simulink model "Simulink"  (R2021a)
settings: Solver=FixedStepAuto  StartTime=0.0  StopTime=10.0  FixedStep=1e-3  RelTol=1e-3  EnableMultiTasking=on
undefined symbols (not defined in the file): D0, D1, D10, D11, D12, D13, D2, D3, D4, D5, D6, D7, D8, D9, PTA0, PTA1, PTA2, PTB23, PTB9, PTC16, PTC17, PTC2, PTC3, PTC4, PTD0, PTD1, PTD2, PTD3
libraries: frdmk64flib x19
settings Model: EnablePacing=on  PacingRate=0.250000  ExtModeTrigDuration=5  Creator=Arun Mistry  LastModifiedBy=Arun Mistry
settings OptimizationCC: EnhancedBackFolding=on  PassReuseOutputArgsAs=Individual arguments  ZeroExternalMemoryAtStartup=off  ZeroInternalMemoryAtStartup=off  MaxStackSize=64  OptimizeBlockOrder=speed  DifferentSizesBufferReuse=on  OptimizationCustomize=off  EfficientTunableParamExpr=on
settings DebuggingCC: ParameterTunabilityLossMsg=error
settings HardwareCC: ProdBitPerPointer=32  ProdBitPerSizeT=32  ProdBitPerPtrDiffT=32  ProdLargestAtomicInteger=Long  ProdLargestAtomicFloat=Double  ProdWordSize=32  ProdHWDeviceType=ARM Compatible->ARM Cortex
settings SFSimCC: MATLABDynamicMemAlloc=off
settings RTWCC: SystemTargetFile=ert.tlc  HardwareBoard=NXP FRDM-K64F  TLCOptions="-aInlineSetEventsForThisBaseRateFcn=TLC_FALSE -aSuppressMultiTaskScheduler=TLC_FALSE  -aRateBasedStepFcn=0"  TemplateMakefile=ert_default_tmf  Toolchain=GNU Tools for ARM Embedded Processors
settings CodeAppCC: ForceParamTrailComments=on  IgnoreCustomStorageClasses=off  OperatorAnnotations=on  SimulinkDataObjDesc=on  SFDataObjDesc=on  InsertBlockDesc=on
settings ERTTargetCC: ExtModeTransport=4  ExtModeMexFile=sendToCommService

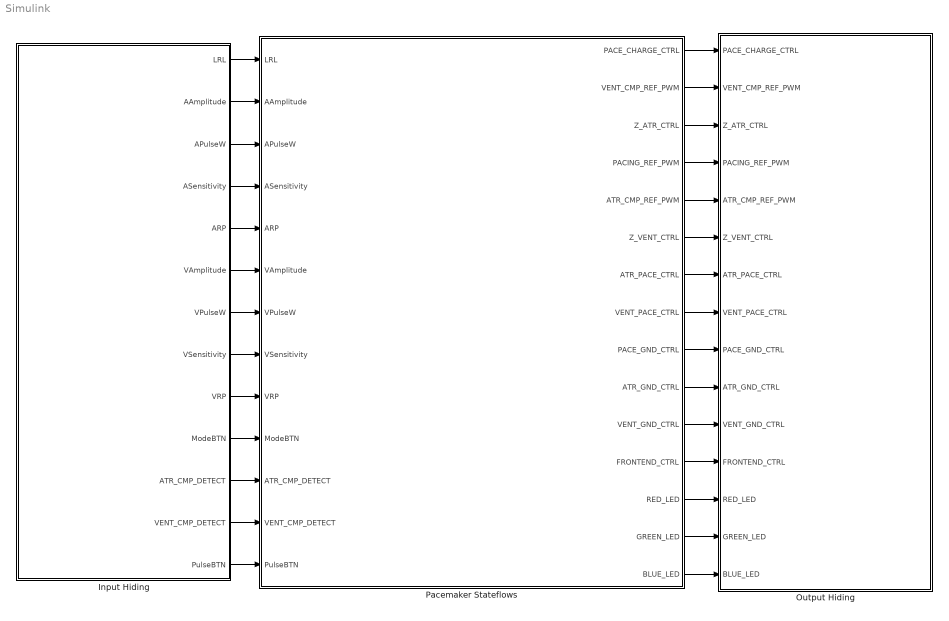
== system Simulink ==
  Input Hiding : Subsystem
  Output Hiding : Subsystem
  Pacemaker Stateflows : Stateflow chart  TreatAsAtomicUnit=on
  wires:
  Input Hiding/13(PulseBTN) -> Pacemaker Stateflows/13(PulseBTN)
  Pacemaker Stateflows/1(PACE_CHARGE_CTRL) -> Output Hiding/1(PACE_CHARGE_CTRL)
  Input Hiding/11(ATR_CMP_DETECT) -> Pacemaker Stateflows/11(ATR_CMP_DETECT)
  Input Hiding/7(VPulseW) -> Pacemaker Stateflows/7(VPulseW)
  Input Hiding/12(VENT_CMP_DETECT) -> Pacemaker Stateflows/12(VENT_CMP_DETECT)
  Pacemaker Stateflows/3(Z_ATR_CTRL) -> Output Hiding/3(Z_ATR_CTRL)
  Input Hiding/3(APulseW) -> Pacemaker Stateflows/3(APulseW)
  Pacemaker Stateflows/7(ATR_PACE_CTRL) -> Output Hiding/7(ATR_PACE_CTRL)
  Pacemaker Stateflows/10(ATR_GND_CTRL) -> Output Hiding/10(ATR_GND_CTRL)
  Input Hiding/10(ModeBTN) -> Pacemaker Stateflows/10(ModeBTN)
  Input Hiding/2(AAmplitude) -> Pacemaker Stateflows/2(AAmplitude)
  Input Hiding/6(VAmplitude) -> Pacemaker Stateflows/6(VAmplitude)
  Pacemaker Stateflows/6(Z_VENT_CTRL) -> Output Hiding/6(Z_VENT_CTRL)
  Pacemaker Stateflows/4(PACING_REF_PWM) -> Output Hiding/4(PACING_REF_PWM)
  Pacemaker Stateflows/11(VENT_GND_CTRL) -> Output Hiding/11(VENT_GND_CTRL)
  Pacemaker Stateflows/9(PACE_GND_CTRL) -> Output Hiding/9(PACE_GND_CTRL)
  Pacemaker Stateflows/8(VENT_PACE_CTRL) -> Output Hiding/8(VENT_PACE_CTRL)
  Input Hiding/1(LRL) -> Pacemaker Stateflows/1(LRL)
  Pacemaker Stateflows/15(BLUE_LED) -> Output Hiding/15(BLUE_LED)
  Input Hiding/4(ASensitivity) -> Pacemaker Stateflows/4(ASensitivity)
  Pacemaker Stateflows/12(FRONTEND_CTRL) -> Output Hiding/12(FRONTEND_CTRL)
  Input Hiding/9(VRP) -> Pacemaker Stateflows/9(VRP)
  Input Hiding/8(VSensitivity) -> Pacemaker Stateflows/8(VSensitivity)
  Input Hiding/5(ARP) -> Pacemaker Stateflows/5(ARP)
  Pacemaker Stateflows/14(GREEN_LED) -> Output Hiding/14(GREEN_LED)
  Pacemaker Stateflows/13(RED_LED) -> Output Hiding/13(RED_LED)
  Pacemaker Stateflows/5(ATR_CMP_REF_PWM) -> Output Hiding/5(ATR_CMP_REF_PWM)
  Pacemaker Stateflows/2(VENT_CMP_REF_PWM) -> Output Hiding/2(VENT_CMP_REF_PWM)

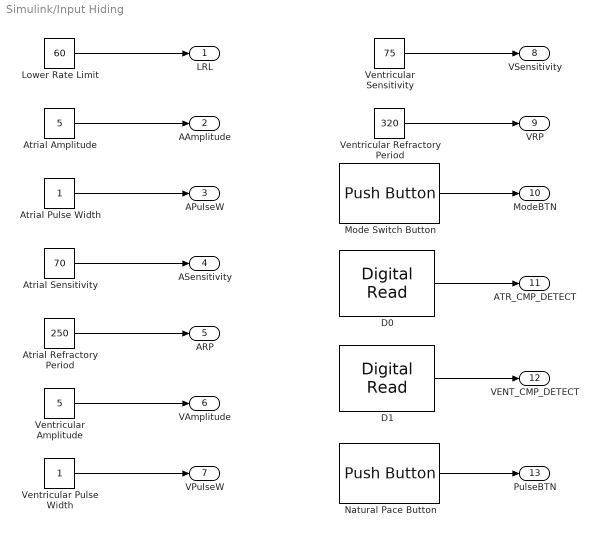
== system Simulink/Input Hiding ==
  Atrial Amplitude : Constant  Value=5  OutDataTypeStr=double
  Atrial Pulse Width : Constant  OutDataTypeStr=double
  Atrial Refractory Period : Constant  Value=250  OutDataTypeStr=double
  Atrial Sensitivity : Constant  Value=70  OutDataTypeStr=double
  D0 : frdmk64flib/Digital Read  Whichpin=PTC16 (D0)  SampleTime=-1
  D1 : frdmk64flib/Digital Read  Whichpin=PTC17 (D1)  SampleTime=-1
  Lower Rate Limit : Constant  Value=60  OutDataTypeStr=double
  Mode Switch Button : frdmk64flib/Push Button  Whichswitch=SW2  SampleTime1=-1
  Natural Pace Button : frdmk64flib/Push Button  Whichswitch=SW3  SampleTime1=-1
  Ventricular Amplitude : Constant  Value=5  OutDataTypeStr=double
  Ventricular Pulse Width : Constant  OutDataTypeStr=double
  Ventricular Refractory Period : Constant  Value=320  OutDataTypeStr=double
  Ventricular Sensitivity : Constant  Value=75  OutDataTypeStr=double
  LRL : Outport  OutDataTypeStr=double
  AAmplitude : Outport  Port=2  OutDataTypeStr=double
  APulseW : Outport  Port=3  OutDataTypeStr=double
  ASensitivity : Outport  Port=4  OutDataTypeStr=double
  ARP : Outport  Port=5  OutDataTypeStr=double
  VAmplitude : Outport  Port=6  OutDataTypeStr=double
  VPulseW : Outport  Port=7  OutDataTypeStr=double
  VSensitivity : Outport  Port=8  OutDataTypeStr=double
  VRP : Outport  Port=9  OutDataTypeStr=double
  ModeBTN : Outport  Port=10  OutDataTypeStr=boolean
  ATR_CMP_DETECT : Outport  Port=11  OutDataTypeStr=boolean
  VENT_CMP_DETECT : Outport  Port=12  OutDataTypeStr=boolean
  PulseBTN : Outport  Port=13  OutDataTypeStr=boolean
  wires:
  Lower Rate Limit/1 -> LRL/1
  Atrial Amplitude/1 -> AAmplitude/1
  Ventricular Amplitude/1 -> VAmplitude/1
  Atrial Pulse Width/1 -> APulseW/1
  Ventricular Pulse Width/1 -> VPulseW/1
  Atrial Sensitivity/1 -> ASensitivity/1
  Ventricular Sensitivity/1 -> VSensitivity/1
  Ventricular Refractory Period/1 -> VRP/1
  Atrial Refractory Period/1 -> ARP/1
  Mode Switch Button/1 -> ModeBTN/1
  Natural Pace Button/1 -> PulseBTN/1
  D0/1 -> ATR_CMP_DETECT/1
  D1/1 -> VENT_CMP_DETECT/1

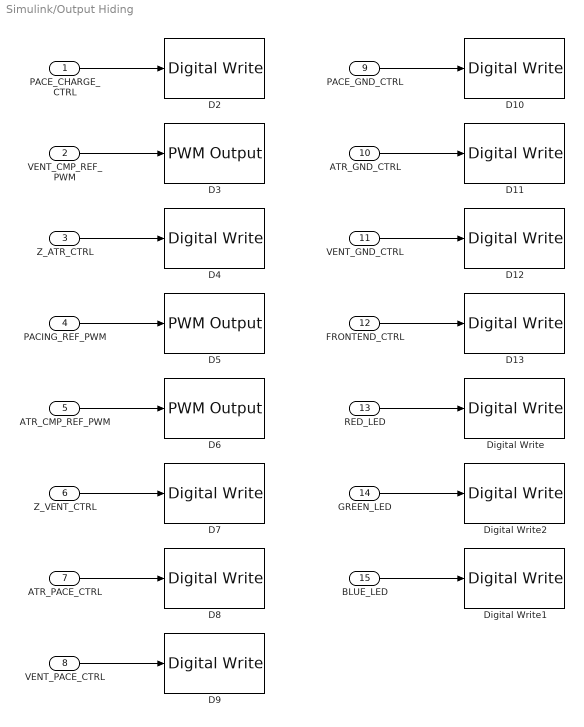
== system Simulink/Output Hiding ==
  PACE_CHARGE_CTRL : Inport  OutDataTypeStr=double
  VENT_CMP_REF_PWM : Inport  Port=2  OutDataTypeStr=double
  Z_ATR_CTRL : Inport  Port=3  OutDataTypeStr=double
  PACING_REF_PWM : Inport  Port=4  OutDataTypeStr=double
  ATR_CMP_REF_PWM : Inport  Port=5  OutDataTypeStr=double
  Z_VENT_CTRL : Inport  Port=6  OutDataTypeStr=double
  ATR_PACE_CTRL : Inport  Port=7  OutDataTypeStr=double
  VENT_PACE_CTRL : Inport  Port=8  OutDataTypeStr=double
  PACE_GND_CTRL : Inport  Port=9  OutDataTypeStr=double
  ATR_GND_CTRL : Inport  Port=10  OutDataTypeStr=double
  VENT_GND_CTRL : Inport  Port=11  OutDataTypeStr=double
  FRONTEND_CTRL : Inport  Port=12  OutDataTypeStr=double
  RED_LED : Inport  Port=13  OutDataTypeStr=double
  GREEN_LED : Inport  Port=14  OutDataTypeStr=double
  BLUE_LED : Inport  Port=15  OutDataTypeStr=double
  D10 : frdmk64flib/Digital Write  Whichpin=PTD0 (D10)
  D11 : frdmk64flib/Digital Write  Whichpin=PTD2 (D11)
  D12 : frdmk64flib/Digital Write  Whichpin=PTD3 (D12)
  D13 : frdmk64flib/Digital Write  Whichpin=PTD1 (D13)
  D2 : frdmk64flib/Digital Write  Whichpin=PTB9 (D2)
  D3 : frdmk64flib/PWM Output  Whichpin=PTA1 (D3)  InitialFrequency=916  InitialDutyCycle=0
  D4 : frdmk64flib/Digital Write  Whichpin=PTB23 (D4)
  D5 : frdmk64flib/PWM Output  Whichpin=PTA2 (D5)  InitialFrequency=2000  InitialDutyCycle=100
  D6 : frdmk64flib/PWM Output  Whichpin=PTC2 (D6)  InitialFrequency=916  InitialDutyCycle=0
  D7 : frdmk64flib/Digital Write  Whichpin=PTC3 (D7)
  "D8 " : frdmk64flib/Digital Write  Whichpin=PTA0 (D8)
  D9 : frdmk64flib/Digital Write  Whichpin=PTC4 (D9)
  Digital Write : frdmk64flib/Digital Write  Whichpin=RED_LED
  Digital Write1 : frdmk64flib/Digital Write  Whichpin=BLUE_LED
  Digital Write2 : frdmk64flib/Digital Write  Whichpin=GREEN_LED
  wires:
  VENT_PACE_CTRL/1 -> D9/1
  ATR_CMP_REF_PWM/1 -> D6/1
  PACE_GND_CTRL/1 -> D10/1
  VENT_CMP_REF_PWM/1 -> D3/1
  PACING_REF_PWM/1 -> D5/1
  ATR_GND_CTRL/1 -> D11/1
  ATR_PACE_CTRL/1 -> "D8 "/1
  PACE_CHARGE_CTRL/1 -> D2/1
  FRONTEND_CTRL/1 -> D13/1
  VENT_GND_CTRL/1 -> D12/1
  Z_ATR_CTRL/1 -> D4/1
  Z_VENT_CTRL/1 -> D7/1
  RED_LED/1 -> Digital Write/1
  BLUE_LED/1 -> Digital Write1/1
  GREEN_LED/1 -> Digital Write2/1

== stateflow chart Simulink/Pacemaker Stateflows ==
  state AOO
    entry:
    VENT_PACE_CTRL = 0; VENT_GND_CTRL = 0; PACE_GND_CTRL = 1;
    Z_VENT_CTRL = 0; Z_ATR_CTRL = 0; PACING_REF_PWM = AAmplitude*20;
    state PACE_ATR
      entry:
      PACE_CHARGE_CTRL = 0;
      ATR_GND_CTRL = 0;
      ATR_PACE_CTRL = 1;
      RED_LED = 1;
    state C22_CHARGE
      entry:
      ATR_PACE_CTRL = 0;
      ATR_GND_CTRL = 1;
      PACE_CHARGE_CTRL = 1;
      RED_LED = 0;
    (default) -> AOO.C22_CHARGE
    AOO.PACE_ATR -> AOO.C22_CHARGE : after(APulseW,msec)
    AOO.C22_CHARGE -> AOO.PACE_ATR : after((60000/LRL)-APulseW,msec)
  state VOO
    entry:
    ATR_PACE_CTRL = 0; ATR_GND_CTRL = 0; PACE_GND_CTRL = 1;
    Z_ATR_CTRL = 0; Z_VENT_CTRL = 0; PACING_REF_PWM = VAmplitude*20;
    state PACE_VENT
      entry:
      PACE_CHARGE_CTRL = 0;
      VENT_GND_CTRL = 0;
      VENT_PACE_CTRL = 1;
      BLUE_LED = 1;
    state C22_CHARGE
      entry:
      VENT_PACE_CTRL = 0;
      VENT_GND_CTRL = 1;
      PACE_CHARGE_CTRL = 1;
      BLUE_LED = 0;
    (default) -> VOO.C22_CHARGE
    VOO.PACE_VENT -> VOO.C22_CHARGE : after(VPulseW,msec)
    VOO.C22_CHARGE -> VOO.PACE_VENT : after((60000/LRL)-VPulseW,msec)
  state MODE
    entry:
    Mode = Mode + 1;
    Mode = rem(Mode ,4);
    RED_LED = 1;
    GREEN_LED = 1;
    BLUE_LED = 1;
    exit:
    RED_LED = 0;
    GREEN_LED = 0;
    BLUE_LED = 0;
  state AAI
    entry:
    VENT_PACE_CTRL = 0; VENT_GND_CTRL = 0; PACE_GND_CTRL = 1;
    Z_VENT_CTRL = 0; Z_ATR_CTRL = 0; FRONTEND_CTRL = 1;
    PACING_REF_PWM = AAmplitude*20; ATR_CMP_REF_PWM=ASensitivity;
    state PACE_ATR
      entry:
      PACE_CHARGE_CTRL = 0;
      ATR_GND_CTRL = 0;
      ATR_PACE_CTRL = 1;
      RED_LED = 1;
    state C22_CHARGE
      entry:
      ATR_PACE_CTRL = 0;
      ATR_GND_CTRL = 1;
      PACE_CHARGE_CTRL = 1;
      RED_LED = 0;
    state REFRACTORY
      entry:
      GREEN_LED = 1;
      exit:
      GREEN_LED = 0;
    (default) -> AAI.C22_CHARGE
    AAI.PACE_ATR -> AAI.C22_CHARGE : [after(APulseW,msec)]
    AAI.C22_CHARGE -> AAI.PACE_ATR [order 2] : after((60000/LRL)-APulseW,msec)
    AAI.REFRACTORY -> AAI.PACE_ATR [order 2] : after(60000/LRL-ARP,msec)
    AAI.C22_CHARGE -> AAI.REFRACTORY [order 1] : after(ARP, msec)
        | [ATR_CMP_DETECT == true || PulseBTN == true]
    AAI.REFRACTORY -> AAI.REFRACTORY [order 1] : after(ARP,msec)[ATR_CMP_DETECT == true || PulseBTN == true]
  state VVI
    entry:
    ATR_PACE_CTRL = 0; ATR_GND_CTRL = 0; PACE_GND_CTRL = 1;
    Z_VENT_CTRL = 0; Z_ATR_CTRL = 0; FRONTEND_CTRL = 1;
    PACING_REF_PWM = VAmplitude*20; VENT_CMP_REF_PWM=VSensitivity;
    state C22_CHARGE
      entry:
      VENT_PACE_CTRL = 0;
      VENT_GND_CTRL = 1;
      PACE_CHARGE_CTRL = 1;
      BLUE_LED = 0;
    state PACE_VENT
      entry:
      PACE_CHARGE_CTRL = 0;
      VENT_GND_CTRL = 0;
      VENT_PACE_CTRL = 1;
      BLUE_LED = 1;
    state REFRACTORY
      entry:
      GREEN_LED = 1;
      exit:
      GREEN_LED = 0;
    (default) -> VVI.C22_CHARGE
    VVI.PACE_VENT -> VVI.C22_CHARGE : [after(VPulseW,msec)]
    VVI.C22_CHARGE -> VVI.PACE_VENT [order 2] : after((60000/LRL)-VPulseW,msec)
    VVI.REFRACTORY -> VVI.PACE_VENT [order 1] : after(60000/LRL-VRP,msec)
    VVI.C22_CHARGE -> VVI.REFRACTORY [order 1] : after(VRP,msec)
        | [VENT_CMP_DETECT == true || PulseBTN == true]
    VVI.REFRACTORY -> VVI.REFRACTORY [order 2] : after(VRP,msec)[VENT_CMP_DETECT == true || PulseBTN == true]
  (default) -> MODE
  MODE -> VOO [order 2] : [Mode == 1 && ModeBTN == false]
  MODE -> AOO [order 1] : [Mode == 0 && ModeBTN == false]
  VOO -> MODE : [ModeBTN == true]
  AOO -> MODE : [ModeBTN == true]
  MODE -> AAI [order 3] : [Mode == 2 && ModeBTN == false]
  AAI -> MODE : [ModeBTN == true]
  VVI -> MODE : [ModeBTN == true]
  MODE -> VVI [order 4] : [Mode == 3 && ModeBTN == false]
  data: LRL input double; AAmplitude input double; APulseW input double; ASensitivity input double; ARP input double; VAmplitude input double; VPulseW input double; VSensitivity input double; VRP input double; PACE_CHARGE_CTRL output double; VENT_CMP_REF_PWM output double; Z_ATR_CTRL output double; PACING_REF_PWM output double; ATR_CMP_REF_PWM output double; Z_VENT_CTRL output double; ATR_PACE_CTRL output double; VENT_PACE_CTRL output double; PACE_GND_CTRL output double; ATR_GND_CTRL output double; VENT_GND_CTRL output double; ModeBTN input boolean; Mode local double =3; FRONTEND_CTRL output double; RED_LED output double; GREEN_LED output double; BLUE_LED output double; ATR_CMP_DETECT input boolean; VENT_CMP_DETECT input boolean; PulseBTN input boolean
